simulink model "tankConPI"  (Simulink 10.1)
settings: Solver=VariableStepAuto  StartTime=0.0  StopTime=10.0  RelTol=1e-3
values from neighbouring files (symbols this model uses):
  a = 1    [tankParams.m]
  Amax = 200    [tankParams.m]
  Amin = 100    [tankParams.m]
  cd = 0.6    [tankParams.m]
  g = 981    [tankParams.m]
  hinit = 10    [tankParams.m]
  hmax = 50    [tankParams.m]
  k = 300    [tankParams.m]
settings Model: Creator=PC  LastModifiedBy=PC
settings DataIOCC: SaveFormat=Dataset  ReturnWorkspaceOutputs=on
settings OptimizationCC: LifeSpan=auto
settings DebuggingCC: UnderspecifiedInitializationDetection=Simplified  MergeDetectMultiDrivingBlocksExec=error  SFUnexpectedBacktrackingDiag=error  SFNoUnconditionalDefaultTransitionDiag=error  SFExecutionAtInitializationDiag=warning  ArithmeticOperatorsInVariantConditions=error
settings HardwareCC: ProdBitPerPointer=64  ProdBitPerSizeT=64  ProdBitPerPtrDiffT=64  ProdLargestAtomicFloat=Float  ProdIntDivRoundTo=Zero  ProdEndianess=LittleEndian  ProdWordSize=64  ProdHWDeviceType=Intel->x86-64 (Windows64)
settings ModelReferenceCC: PropagateSignalLabelsOutOfModel=on
settings SFSimCC: SimUseLocalCustomCode=on  CustomCodeUndefinedFunction=FilterOut
settings RTWCC: RTWUseLocalCustomCode=on
settings CodeAppCC: StateflowObjectComments=off
settings GRTTargetCC: TargetLangStandard=C99 (ISO)  CombineOutputUpdateFcns=on  GRTInterface=off
settings ConfigComp: CovMetricSettings=dwe  CovHtmlReporting=off  CovSaveCumulativeToWorkspaceVar=off  CovSaveSingleToWorkspaceVar=off  CovExternalEMLEnable=on

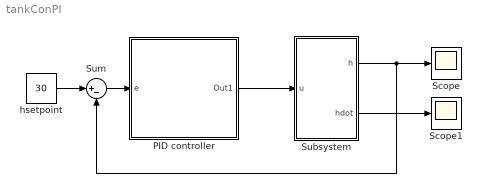
== system tankConPI ==
  PID controller : Subsystem
  Scope : Scope
  Scope1 : Scope
  Subsystem : Subsystem
  Sum : Sum  Inputs=|+-
  hsetpoint : Constant  Value=30
  wires:
  Sum/1 -> PID controller/1(e)
  hsetpoint/1 -> Sum/1
  Subsystem/1(h) -> Sum/2, Scope/1
  Subsystem/2(hdot) -> Scope1/1
  PID controller/1(Out1) -> Subsystem/1(u)

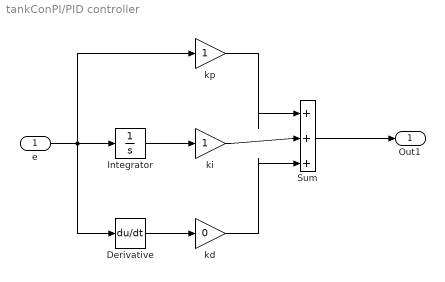
== system tankConPI/PID controller ==
  e : Inport
  Derivative : Derivative
  Integrator : Integrator
  Sum : Sum  Inputs=|+++
  kd : Gain  Gain=0
  ki : Gain
  kp : Gain
  Out1 : Outport
  wires:
  Integrator/1 -> ki/1
  Derivative/1 -> kd/1
  e/1 -> Derivative/1, kp/1, Integrator/1
  kp/1 -> Sum/1
  ki/1 -> Sum/2
  kd/1 -> Sum/3
  Sum/1 -> Out1/1

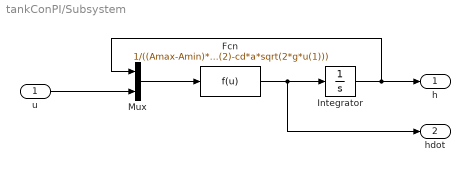
== system tankConPI/Subsystem ==
  u : Inport
  Fcn : Fcn  Expr=1/((Amax-Amin)*u(1)/hmax+Amin)*(k*u(2)-cd*a*sqrt(2*g*u(1)))
  Integrator : Integrator  InitialCondition=hinit
  Mux : Mux  Inputs=2
  h : Outport
  hdot : Outport  Port=2
  wires:
  Mux/1 -> Fcn/1
  Fcn/1 -> hdot/1, Integrator/1
  Integrator/1 -> Mux/1, h/1
  u/1 -> Mux/2
